simulink model "generic"  (R2022b)
settings: Solver=ode45  StartTime=0.0  StopTime=inf  RelTol=1e-3  EnableMultiTasking=on
values from neighbouring files (symbols this model uses):
  A = cell2mat(A_cell)    [MPCController1.m]    (also in MPC_Fmincon.m)
  B = cell2mat(B_cell)    [MPCController1.m]    (also in MPC_Fmincon.m)
  brake_select = ones(length(speed), length(steering_angle))    [TwoDLook_uptable.m]
  curvature = 0.000:0.001:1    [TwoDLook_uptable.m]
  m = 1600    [MPCController1.m]    (also in MPCController2.m; MPC_Fmincon.m)
  speed = 0:0.1:100    [TwoDLook_uptable.m]
undefined symbols (not defined in the file or in its folder): Amplifier, DiscIntNeverNeededParam, K_d_yawrate, K_dsteering, k_speed, k_stanley, kd, ki, kp, path_curvature
libraries: CarMaker4SL x97, simulink x6, cstblocks x6, simulink_extras x4, autolibshared x1, mpcadaslib x1
(part 6 of 6)

== matlab function generic/CarMaker/VehicleControl/CreateBus VhclCtrl1/Stanley steering & speed//Brake controller/Road sensor set & path planning/Road sensor set & path planning/A* star path planning/getInstantaneousPath Function ==
  data: generated_path input; lookahead_distance input; current_position input; instantaneous_points output; current_heading input
function instantaneous_points = getInstantaneousPoint(generated_path, lookahead_distance, current_position, current_heading)
    % Parameters
    num_points = size(generated_path, 2);
    rotated_point = zeros(1,2);
    instantaneous_point= zeros(1,2);
    disp(generated_path)
    % Find the closest point on the generated path to the current position
    distances = sqrt((generated_path(1, :) - current_position(1)).^2 + (generated_path(2, :) - current_position(2)).^2);
    [~, closest_point_index] = min(distances);
     % Extract the last point along the path based on lookahead distance
    cumulative_distances = cumsum(sqrt(diff(generated_path(1, :)).^2 + diff(generated_path(2, :)).^2));
     % Check if cumulative_distances is non-empty
    if all(cumulative_distances == 0)
        % If there is only one point in the path, use that point
        lookahead_index = closest_point_index;
    else
        % Otherwise, find the index based on lookahead distance
        lookahead_index = closest_point_index + find(cumulative_distances >= lookahead_distance, 1, 'first');
    end
    disp(lookahead_index)
    disp('333')
    
    % Ensure lookahead_index is within valid range
    lookahead_index = min(lookahead_index, num_points);
    
    % Extract the last point from the path
    instantaneous_point = generated_path(:, lookahead_index);
    
    % Transform the point to the vehicle's local coordinate system
    delta_x = instantaneous_point(1) - current_position(1);
    delta_y = instantaneous_point(2) - current_position(2);
    
    rotated_point = [cos(-current_heading) -sin(-current_heading); sin(-current_heading) cos(-current_heading)] * [delta_x; delta_y];
    
    % Adjust the rotated point to be relative to the current position
    instantaneous_points = [current_position(1) + rotated_point(1) current_position(2) + rotated_point(2)];
end

== matlab function generic/CarMaker/VehicleControl/CreateBus VhclCtrl1/Stanley steering & speed//Brake controller/Road sensor set & path planning/Road sensor set & path planning/Dijkestra path planning/getInstantaneousPath Function ==
  data: generated_path input; lookahead_distance input; current_position input; instantaneous_points output; current_heading input
function instantaneous_points = getInstantaneousPoint(generated_path, lookahead_distance, current_position, current_heading)
    % Parameters
    num_points = size(generated_path, 2);
    rotated_point = zeros(1,2);
    instantaneous_point= zeros(1,2);
    disp(generated_path)
    % Find the closest point on the generated path to the current position
    distances = sqrt((generated_path(1, :) - current_position(1)).^2 + (generated_path(2, :) - current_position(2)).^2);
    [~, closest_point_index] = min(distances);
     % Extract the last point along the path based on lookahead distance
    cumulative_distances = cumsum(sqrt(diff(generated_path(1, :)).^2 + diff(generated_path(2, :)).^2));
     % Check if cumulative_distances is non-empty
    if all(cumulative_distances == 0)
        % If there is only one point in the path, use that point
        lookahead_index = closest_point_index;
    else
        % Otherwise, find the index based on lookahead distance
        lookahead_index = closest_point_index + find(cumulative_distances >= lookahead_distance, 1, 'first');
    end
    disp(lookahead_index)
    disp('333')
    
    % Ensure lookahead_index is within valid range
    lookahead_index = min(lookahead_index, num_points);
    
    % Extract the last point from the path
    instantaneous_point = generated_path(:, lookahead_index);
    
    % Transform the point to the vehicle's local coordinate system
    delta_x = instantaneous_point(1) - current_position(1);
    delta_y = instantaneous_point(2) - current_position(2);
    
    rotated_point = [cos(-current_heading) -sin(-current_heading); sin(-current_heading) cos(-current_heading)] * [delta_x; delta_y];
    
    % Adjust the rotated point to be relative to the current position
    instantaneous_points = [current_position(1) + rotated_point(1) current_position(2) + rotated_point(2)];
end

== matlab function generic/CarMaker/VehicleControl/CreateBus VhclCtrl1/Stanley steering & speed//Brake controller/Stanley_controller_with_thottle_and_brake_commands/Stanley steering + PID speed controller/Speed_controller/advancedPID_speed_and_brake_control ==
  settings: updateMethod=DISCRETE
  data: path_curv input; throttle output; min_s_speed input; brake_cmd output; speed_act input; desired_speed input; Kd_speed input; Ki_speed input; Kp_speed input
function [throttle, brake_cmd] = advanced_speed_and_brake_control(path_curv, min_s_speed, speed_act, desired_speed,Kd_speed,Ki_speed,Kp_speed)
    persistent integrator_speed;
    persistent prev_speed_error;
    persistent integrator_brake;
    persistent prev_brake_error;

    if isempty(integrator_speed)
        integrator_speed = 0;
        prev_speed_error = 0;
        integrator_brake = 0;
        prev_brake_error = 0;
    end


   
    % Speed Control (PID)
    %disp(speed_act)
    %disp("teh speed is ")
    %disp(desired_speed)
    speed_error = desired_speed - speed_act;
    %Kp_speed = 1.900;
    %Ki_speed = 0.0300;
    %Kd_speed = 1.00;
    integrator_speed = integrator_speed + speed_error;
    derivative_speed = speed_error - prev_speed_error;
    
    throttle = Kp_speed * speed_error + Ki_speed * integrator_speed + Kd_speed * derivative_speed;

    % Braking Control (PID)
    brake_error = -speed_error;
    Kp_brake = 0.05;
    Ki_brake = 0.01;
    Kd_brake = 0.05;
    integrator_brake = integrator_brake + brake_error;
    derivative_brake = brake_error - prev_brake_error;
    brake_cmd = Kp_brake * brake_error + Ki_brake * integrator_brake + Kd_brake * derivative_brake;

    % Predictive Braking based on Path Curvature
    path_curvature = max(path_curv);
    min_safe_speed = max(min_s_speed);
    predictive_brake_factor = speed_act/100;
    if path_curvature > 0 && speed_act < min_safe_speed
        brake_cmd = brake_cmd + predictive_brake_factor * (min_safe_speed - speed_act);
    end
    % Update persistent variables
    prev_speed_error = speed_error;
    prev_brake_error = brake_error;
end

== matlab function generic/CarMaker/VehicleControl/CreateBus VhclCtrl1/Stanley steering & speed//Brake controller/Stanley_controller_with_thottle_and_brake_commands/MPCLongitudianl_contorl/Speed_regulator/MATLAB Function ==
  data: speed input; braking_distance output; others output
function [braking_distance,others]= calculateBrakingDistance(speed)
    % Estimate the braking distance
        max_deceleration = 5.0;
        safety_factor = 1.5;
        braking_distance = (speed^2) / (2 * max_deceleration) * safety_factor;
        others = speed^2 *3.6/(250*1)* safety_factor*2.2;
end

== matlab function generic/CarMaker/VehicleControl/CreateBus VhclCtrl1/MPC_steering_controllers/Subsystem/MATLAB Function2 ==
  data: heading_error input; dt input; yaw_angle input; yaw_rate input; vx input; delta output; vy input; reference_trajectory input; x input; u input
function delta = adaptive_steering_mpc( heading_error,dt,yaw_angle,yaw_rate, vx, vy, reference_trajectory,x,u)
    % Adaptive Model Predictive Controller (Adaptive MPC) for steering control
    function [c, ceq] = nonlinear_constraints(u, x, vx, dt)
    % Extract control input
    %steering_angle = u(1);
    longitudinal_velocity = u(2);

        % Calculate the next state based on the system dynamics
        x_next = calculate_dynamics(x, u, m, cf, cr, lf, lr, dt, vx);
    
        % Enforce constraints
        c1 = x_next(1) - x(1) - vx * cos(x(4)) * dt;  % Constraint for x position
        c2 = x_next(2) - x(2) - vx * sin(x(4)) * dt;  % Constraint for y position
        
        c3 = x_next(4) - x(4) - longitudinal_velocity * dt;  % Constraint for yaw angle
        c4 = -x(2) - vx * sin(x(4)) * dt;  % Ensure lateral position is within bounds
    
        % Combine inequality constraints
        c = [c1; c2; c3; c4];
    
        % No equality constraints (ceq = 0)
        ceq = [];
    end
        function J = cost_function(u, x, Q, R, N, dt, m, cf, cr, lf, lr, vx, vy)
        % Cost function for fmincon
        x_pred = predict_states(x, u, m, cf, cr, lf, lr, dt, N, vx);
        J = (x_pred - reference_state)' * Q * (x_pred - reference_state) + u' * R * u;
        
    end

    function x_pred = predict_states(x, u, m, cf, cr, lf, lr, dt, N, vx)
        % Predict future states using the model
        A = calculate_A(x, u, m, cf, cr, lf, lr, vx);
        B = calculate_B(x, u, m, cf, cr, lf, lr, vx);

        x_pred = x;
        for i = 1:N
            x_pred = x_pred + A * x_pred * dt + B * u * dt;
        end
    end

    function A = calculate_A(x, u, m, cf, cr, lf, lr, vx)
        % Calculate state matrix A
        A = [-((cf + cr) / (m * vx)), -vx - ((cf * lf - cr * lr) / (m * vx^2)), 0, 0;
             -((cf * lf - cr * lr) / (m * vx)), -((cf * lf^2 + cr * lr^2) / (m * vx^2)), 0, 0;
             1, 0, 0, vx;
             0, 1, vx, 0];
    end

    function B = calculate_B(x, u, m, cf, cr, lf, lr, vx)
        % Calculate input matrix B
        B = [2 * cf / m, 0;
             2 * cf * lf / (m * vx), 0;
             0, 1;
             0, (2 * lf * cf - 2 * lr * cr) / (m * vx)];
    end

    function x_next = calculate_dynamics(x, u, m, cf, cr, lf, lr, dt, vx)
        % Calculate next state using the model
        A = calculate_A(x, u, m, cf, cr, lf, lr, vx);
        B = calculate_B(x, u, m, cf, cr, lf, lr, vx);

        x_next = x + (A * x + B * u) * dt;
    end
    % Define MPC parameters (modify as needed)
    N = 5;  % Prediction horizon
    Q = diag([1, 1, 1, 1]);  % State cost matrix (including heading error)
    R = diag([0.1, 0.1]);  % Input cost matrix

    % Define system parameters (replace these with your actual vehicle parameters)
    m = 1600;           % Vehicle mass [kg]
    l = 2.975;          % Wheelbase [m]
    Iz = 2986.624;      % Vehicle inertia [kg*m^2]
    cf = 80000;         % Front tire cornering stiffness [N/rad]
    cr = 120000;        % Rear tire cornering stiffness [N/rad]
    lf = 1.5;           % Distance from center of gravity to front axle [m]
    lr = 1.475;         % Distance from center of gravity to rear axle [m]

    % Adaptive parameters
    alpha = 0.1;  % Adaptation rate
    theta = [0.1; 0.1];  % Initial guess of parameters

    % State vector (simplified, assuming heading_error is the heading error)
    x = [heading_error; 0; 0; 0];  % Adding lateral error and lateral velocity to the state vector


    % Reference trajectory
    %reference_index = 1;  % Choose the appropriate index for the current time step
    % Extract x and y positions from the trajectory at the chosen index
    x_position = reference_trajectory(1,:);
    y_position = reference_trajectory(2,:);
    % Construct the reference_state vector
    reference_state = [y_position; yaw_angle; vy; yaw_rate];

    % Define cost and constraints for fmincon
    costFunction = @(u) cost_function(u, x, Q, R, N, dt, m, cf, cr, lf, lr, vx, vy);
    lb = [-1.6; -30];  % Lower bounds on steering input and longitudinal velocity change
    ub = [1.6; 30];    % Upper bounds on steering input and longitudinal velocity change
    u0 = [0.1; 0.1];  % Initial guess
    nonlcon = @(u) nonlinear_constraints(u, x, vx, dt);
    % Solve optimization problem to get optimal steering input
    options = optimoptions('fmincon', 'Display', 'off', 'Algorithm', 'sqp');
    %u_opt = fmincon(costFunction, u0, [], [], [], [], lb, ub, [], options);
    disp(reference_state)
    disp(cost_function(u, x, Q, R, N, dt, m, cf, cr, lf, lr, vx, vy))
    u_opt = fmincon(costFunction, u0, [], [], [], [], lb, ub, nonlcon, options);
    % Extract control input (steering angle and longitudinal velocity change)
    delta = u_opt(1);

    % Update adaptive parameters online (using a simple gradient descent)
    %x_next = calculate_dynamics(x, u_opt, m, cf, cr, lf, lr, dt, vx, vy);
    %theta = theta - alpha * (x_next - x) * x';


end

== matlab function generic/CarMaker/VehicleControl/CreateBus VhclCtrl1/MPC_steering_controllers/Subsystem/MATLAB Function6 ==
  data: current_heading input; dt input; vx input; delta output; vy input
function delta = adaptive_steering_mpc(current_heading, dt, vx, vy)
    % Adaptive Model Predictive Controller (Adaptive MPC) for steering control
    persistent model_params theta
        
    function params = initialize_model_params(m, lf, lr, Iz)
        % Initialize model parameters
        % Define the state-space model
        A = [-2 * (lf + lr) / (m * vx), -vx - 2 * (lf * cf - lr * cr) / (m * vx);
             -2 * (lf * cf - lr * cr) / Iz, -2 * (lf^2 * cf + lr^2 * cr) / Iz];
    
        B = [2 * cf / m; 2 * lf * cf / Iz];
    
        % Store parameters in a struct
        params.A = A;
        params.B = B;
    end
    
    function dx = calculate_dynamics(u, params, vx, vy)
        % Calculate the dynamics of the system (Bicycle Model)
    
        % Unpack state variables
        vy1 = vy - params.B(2) * u;  % Correct lateral velocity for the tire slip angle
    
        % Bicycle model equations
        a = (2 * (u - vy1)) / (params.A(1, 2) * vx);
        b = (2 * lf * (u - vy1)) / params.A(2, 2);
    
        % State dynamics
        dx1 = a * dt;
        dx2 = b * dt;
    
        % Update state variables
        dx = [dx1; dx2];
    end

    % Define Q and R matrices
    Q = eye(2);  % Weighting matrix for state
    R = eye(1);  % Weighting matrix for control input

    % Define system parameters (replace these with your actual vehicle parameters)
    m = 1600;           % Vehicle mass [kg]
    l = 2.975;          % Wheelbase [m]
    Iz = 2986.624;      % Vehicle inertia [kg*m^2]
    cf = 80000;         % Front tire cornering stiffness [N/rad]
    cr = 120000;        % Rear tire cornering stiffness [N/rad]
    lf = 1.5;           % Distance from center of gravity to front axle [m]
    lr = 1.475;         % Distance from center of gravity to rear axle [m]

    % Adaptive parameters
    alpha = 0.1;  % Adaptation rate

    % Update the model parameters if not initialized
    if isempty(model_params)
        model_params = initialize_model_params(m, lf, lr, Iz);
    end

    % Update adaptive parameters if not initialized
    if isempty(theta)
        theta = [0.1; 0.1];  % Initial guess of parameters
    end

    % State vector (simplified, assuming current_heading is the heading error)
    x = [current_heading; 0];

    % Define matrices for quadprog
    H = blkdiag(Q, R);
    f = zeros(size(H, 1), 1);

    % Define linear inequality constraints for quadprog
    Aineq = [];
    Bineq = [];
    % Define linear equality constraints for quadprog
    Aeq = [];
    Beq = [];
    % Define lower and upper bounds for quadprog
    lb = [-1.6; -1.6; -1.6];  % Lower bounds on steering input for each dimension
    ub = [1.6; 1.6; 1.6];     % Upper bounds on steering input for each dimension


    % Initial guess for the control input
    u0 = zeros(size(H, 2), 1);  % Initialize u0 with the correct size

    % Solve the quadratic programming problem with quadprog
    options = optimoptions('quadprog', 'Display', 'off','Algorithm','active-set');
    [u_opt, ~, exitflag] = quadprog(H, f, Aineq, Bineq, Aeq, Beq, lb, ub, u0, options);

    % Check if optimization was successful
    if exitflag <= 0
        error('Quadprog failed to converge. Consider adjusting the problem formulation or solver options.');
    end

    % Update adaptive parameters online (using a simple gradient descent)
    %x_next = x + calculate_dynamics(u_opt, model_params, vx, vy);
    %theta = theta - alpha * (x_next - (x + calculate_dynamics(u_opt, model_params, vx, vy))) * x';

    % Extract control input (steering angle) from the optimization result
    delta = u_opt;
end

== matlab function generic/CarMaker/VehicleControl/CreateBus VhclCtrl1/MPC_steering_controllers/Subsystem/MATLAB Function7 ==
  data: u input; dt input; vx input; delta output; vy input; cr input; cf input; yaw input; dx output; dx1 output
function [delta,dx,dx1] = adaptive_steering_mpc(u, dt, vx, vy,cr,cf,yaw)
    % Adaptive Model Predictive Controller (Adaptive MPC) for steering control
   % persistent model_params theta
    % Define Q and R matrices
    Q = eye(2);  % Weighting matrix for state
    R = eye(1);  % Weighting matrix for control input

    % Define system parameters (replace these with your actual vehicle parameters)
    m = 1600;           % Vehicle mass [kg]
    l = 2.975;          % Wheelbase [m]
    Iz = 2986.624;      % Vehicle inertia [kg*m^2]
    %cf = 80000;         % Front tire cornering stiffness [N/rad]
    %cr = 120000;        % Rear tire cornering stiffness [N/rad]
    lf = 1.488;           % Distance from center of gravity to front axle [m]
    lr = -1.487;         % Distance from center of gravity to rear axle [m]
    if vx<0.5
        vx = 0.5;
    end
    function params = initialize_model_params(Iz,m,vx,cf,cr ,lf, lr)
        % Initialize model parameters
        % Define the state-space model
        A = [-(cr + cf) / (m * vx), -(lf * cf - lr * cr) / (m * vx)+vx^2;
             -(lf * cf - lr * cr) / (Iz*vx), -(lf^2 * cf + lr^2 * cr) / (Iz*vx)];
    
        B = [cf / m, cr/m; lf * cf / Iz, -lr*cr/Iz];
    
        % Store parameters in a struct
        params.A = A;
        params.B = B;
    end
    
    function [dx,dx1] = calculate_dynamics(params, yaw, vy,lf,dt,u)
        % Calculate the dynamics of the system (Bicycle Model)
    
        % Unpack state variables
        vy1 = vy - params.B(2) * u(1);  % Correct lateral velocity for the tire slip angle
        %vy1 = params.B(2);
        % Bicycle model equations
        %a = (2 * (u(1) - vy1)) / (params.A(1, 2) * vx);
        %b = (2 * lf * (u(2) - vy1)) / params.A(2, 2);
        % State dynamics
        %dx1 = a * dt;
        %dx2 = b * dt;
        dx1 = params.B *[0;u(2)]*dt;
        x_dot = params.A *[vy1;yaw]*dt+params.B *[0;u(2)]*dt;
        % Update state variables
        dx =x_dot; %[dx1; dx2];
    end
    params = initialize_model_params(Iz,m,vx,cf,cr ,lf, lr);
    [dx,dx1] = calculate_dynamics(params, yaw, vy,lf,dt,u);
    delta = atan(dx(2)*l/(vx*(1+ (-0.01*vx))));

%     % Adaptive parameters
%     alpha = 0.1;  % Adaptation rate
% 
%     % Update the model parameters if not initialized
%     if isempty(model_params)
%         model_params = initialize_model_params(m, lf, lr, Iz);
%     end
% 
%     % Update adaptive parameters if not initialized
%     if isempty(theta)
%         theta = [0.1; 0.1];  % Initial guess of parameters
%     end
% 
%     % State vector (simplified, assuming current_heading is the heading error)
%     x = [current_heading; 0];
% 
%     % Define matrices for quadprog
%     H = blkdiag(Q, R);
%     f = zeros(size(H, 1), 1);
% 
%     % Define linear inequality constraints for quadprog
%     Aineq = [];
%     Bineq = [];
%     % Define linear equality constraints for quadprog
%     Aeq = [];
%     Beq = [];
%     % Define lower and upper bounds for quadprog
%     lb = [-1.6; -1.6; -1.6];  % Lower bounds on steering input for each dimension
%     ub = [1.6; 1.6; 1.6];     % Upper bounds on steering input for each dimension
% 
% 
%     % Initial guess for the control input
%     u0 = zeros(size(H, 2), 1);  % Initialize u0 with the correct size
% 
%     % Solve the quadratic programming problem with quadprog
%     options = optimoptions('quadprog', 'Display', 'off','Algorithm','active-set');
%     [u_opt, ~, exitflag] = quadprog(H, f, Aineq, Bineq, Aeq, Beq, lb, ub, u0, options);
% 
%     % Check if optimization was successful
%     if exitflag <= 0
%         error('Quadprog failed to converge. Consider adjusting the problem formulation or solver options.');
%     end
% 
%     % Update adaptive parameters online (using a simple gradient descent)
%     %x_next = x + calculate_dynamics(u_opt, model_params, vx, vy);
%     %theta = theta - alpha * (x_next - (x + calculate_dynamics(u_opt, model_params, vx, vy))) * x';
% 
%     % Extract control input (steering angle) from the optimization result
%     delta = u_opt;
end

== matlab function generic/CarMaker/VehicleControl/CreateBus VhclCtrl1/MPC_steering_controllers/Tradition_MPC/MPC_steering_control ==
  data: Lateral_deviation input; steering_cmd output; A input; B input
function steering_cmd = MPC_Steering_control(Lateral_deviation,A,B)
    % Model Predictive Controller (MPC) for speed contol
    %speed_ref  = speed_rf+0.4;
    %Lateral_deviation= current_speed - speed_ref;
    % Define MPC parameters
    Ts = 0.1;  % Sampling time
    N = 10;    % Prediction horizon
    Q = 1;     % State weight
    R = 1;     % Input weight
    S = 0.1;   % Terminal state weight (integral term)
    
    % State-space model (simplified for illustration)
    %A = 0.8;
    %B = Ts;
    
    % Define cost and constraints for fmincon
    costFunction = @(u) (Lateral_deviation + B * u)' * Q * (Lateral_deviation + B * u) + u' * R * u + S * sum(u);
    Aeq = [];
    Beq = [];
    Aineq = [];
    Bineq = [];
    lb = -1.6; % Lower bound on throttle_Brake
    ub = 1.6;  % Upper bound on throttle_Brake
    
    % Steady-state error constraint
    Aineq = [Aineq; B];
    Bineq = [Bineq; -Lateral_deviation];
    
    % Initial guess
    u0 = 0;
    
    % Solve optimization problem
    options = optimoptions('fmincon', 'Display', 'off', 'Algorithm', 'sqp');
    u_opt = fmincon(costFunction, u0, Aineq, Bineq, Aeq, Beq, lb, ub, [], options);
    
    % Extract control input (throttle_Brake) from the optimization result
    steering_cmd = u_opt;
end

== matlab function generic/CarMaker/VehicleControl/CreateBus VhclCtrl1/MPC_steering_controllers/Tradition_MPC/MPC_steering_control1 ==
  data: Heading_error input; steering_cmd output; A input; B input
function steering_cmd = MPC_Steering_control(Heading_error,A,B)
    % Model Predictive Controller (MPC) for speed contol
    %speed_ref  = speed_rf+0.4;
    %Heading_error= current_speed - speed_ref;
    % Define MPC parameters
    Ts = 0.1;  % Sampling time
    N = 10;    % Prediction horizon
    Q = 1;     % State weight
    R = 1;     % Input weight
    S = 0.1;   % Terminal state weight (integral term)
    
    % State-space model (simplified for illustration)
    %A = 0.8;
    %B = Ts;
    
    % Define cost and constraints for fmincon
    costFunction = @(u) (Heading_error + B * u)' * Q * (Heading_error + B * u) + u' * R * u + S * sum(u);
    Aeq = [];
    Beq = [];
    Aineq = [];
    Bineq = [];
    lb = -1.6; % Lower bound on throttle_Brake
    ub = 1.6;  % Upper bound on throttle_Brake
    
    % Steady-state error constraint
    Aineq = [Aineq; B];
    Bineq = [Bineq; -Heading_error];
    
    % Initial guess
    u0 = 0;
    
    % Solve optimization problem
    options = optimoptions('fmincon', 'Display', 'off', 'Algorithm', 'sqp');
    u_opt = fmincon(costFunction, u0, Aineq, Bineq, Aeq, Beq, lb, ub, [], options);
    
    % Extract control input (throttle_Brake) from the optimization result
    steering_cmd = u_opt;
end

== matlab function generic/CarMaker/VehicleControl/CreateBus VhclCtrl1/Stanley steering & speed//Brake controller/Stanley_controller_with_thottle_and_brake_commands/MPCLongitudianl_contorl/MPC_speed_control ==
  data: speed_error input; throttle_Brake output; A input; B input
function throttle_Brake = MPC_speed_control(speed_error,A,B)
    % Model Predictive Controller (MPC) for speed contol
    %speed_ref  = speed_rf+0.4;
    %speed_error= current_speed - speed_ref;
    % Define MPC parameters
    Ts = 0.1;  % Sampling time
    N = 10;    % Prediction horizon
    Q = 1;     % State weight
    R = 1;     % Input weight
    S = 0.1;   % Terminal state weight (integral term)
    
    % State-space model (simplified for illustration)
    %A = 0.8;
    %B = Ts;
    
    % Define cost and constraints for fmincon
    costFunction = @(u) (speed_error + B * u)' * Q * (speed_error + B * u) + u' * R * u + S * sum(u);
    Aeq = [];
    Beq = [];
    Aineq = [];
    Bineq = [];
    lb = 0; % Lower bound on throttle_Brake
    ub = 1;  % Upper bound on throttle_Brake
    
    % Steady-state error constraint
    Aineq = [Aineq; B];
    Bineq = [Bineq; -speed_error];
    
    % Initial guess
    u0 = 0;
    
    % Solve optimization problem
    options = optimoptions('fmincon', 'Display', 'off', 'Algorithm', 'sqp');
    u_opt = fmincon(costFunction, u0, Aineq, Bineq, Aeq, Beq, lb, ub, [], options);
    
    % Extract control input (throttle_Brake) from the optimization result
    throttle_Brake = u_opt;
end

== matlab function generic/CarMaker/VehicleControl/CreateBus VhclCtrl1/Stanley steering & speed//Brake controller/Stanley controller with path_planning/Stanley controller with path_planning/MATLAB Function ==
  data: path input; dev input; e output; yaw input; speed_act input; err_fr_axle output; cross_track_steering output; heading_err output; steering output
function [e, err_fr_axle, cross_track_steering, heading_err, steering]  = conversion(path,dev,yaw,speed_act)
%path = [path_x;path_y];
function distance = calc_distance(pt,v1,v2)
    vect = v1 - v2;
    p_to_vect = pt - v2;
    crossVP = cross(vect,p_to_vect);
    distance = norm(crossVP) / norm(vect) * crossVP(3)/abs(crossVP(3));
end

e = zeros(1);
cross_track_steering = zeros(1);
heading_err = zeros(1);
steering=zeros(1);
err_fr_axle = zeros(1);

k_exp = 1.3059;
k = 15.028 + speed_act^k_exp;
k_ref = 2.62;

% path_index = fix(k_path * speed_act);
% if path_index > 13
%     path_index = 13;
% end
% 
% P_prev = path(:,6 + path_index);
% P_next = path(:,7 + path_index);

fr_axle = [-1.488 0 0];
distances = sqrt((path(1,:) - 1.488).^2 + (path(2,:) - 0).^2);
% Find the index of the closest point on the path
[~,err_fr_axle_ind] = min(distances);
if err_fr_axle_ind == 1
    err_fr_axle_ind = 2;
end
err_fr_axle = calc_distance(fr_axle,[path(1,err_fr_axle_ind - 1) path(2,err_fr_axle_ind - 1) 0],[path(1,err_fr_axle_ind) path(2,err_fr_axle_ind) 0]);

B = [-1.488 + k_ref * (speed_act / 27) 0 0];
distances_err = sqrt((path(1,:) - B(1)).^2 + (path(2,:) - 0).^2);
[~,err_ind] = min(distances_err);
if err_ind < 2
    err_ind = 2;
end
error = calc_distance(B,[path(1,err_ind - 1) path(2,err_ind - 1) 0],[path(1,err_ind) path(2,err_ind) 0]);


P_prev = path(:, err_ind-1);
P_next = path(:, err_ind);

x1 = P_prev(1,1);
y1 = P_prev(2,1);
x2 = P_next(1,1);
y2 = P_next(2,1);

a = (y2 - y1)/-(x2 + x1);
b = 1;
%c = -x1 * (y2 - y1) + y1 * (x2 - x1);


if speed_act ~= 0
    %e = c+b*y1/sqrt((a^2)+(b^2));
    e = error;
    
    cross_track_steering = atan(k * e / speed_act);
    heading_err = atan(-a / b) - yaw;
    %heading_err = 1/(tan(-a/b))-yaw;
    steering = heading_err + cross_track_steering;
end
end

== matlab function generic/CarMaker/VehicleControl/CreateBus VhclCtrl1/MPC_steering_controllers/Subsystem/MATLAB Function1 ==
  data: dev input; steering output; B input
function steering = advanced_speed_control_mpc(dev,B)
    % Model Predictive Controller (MPC) for speed contol
    % Define MPC parameters
    Ts = 0.1;  % Sampling time
    N = 10;    % Prediction horizon
    Q = 1;     % State weight
    R = 1;     % Input weight
    S = 0.1;   % Terminal state weight (integral term)
    
    % State-space model (simplified for illustration)
    %A = 0.8;
    %B = Ts;
    
    % Define cost and constraints for fmincon
    costFunction = @(u) (dev + B * u)' * Q * (dev + B * u) + u' * R * u + S * sum(u);
    Aeq = [];
    Beq = [];
    Aineq = [];
    Bineq = [];
    lb = -3.14; % Lower bound on throttle
    ub = 3.14;  % Upper bound on throttle
    
    % Steady-state error constraint
    Aineq = [Aineq; B];
    Bineq = [Bineq; -dev];
    
    % Initial guess
    u0 = 0;
    
    % Solve optimization problem
    options = optimoptions('fmincon', 'Display', 'off', 'Algorithm', 'sqp');
    u_opt = fmincon(costFunction, u0, Aineq, Bineq, Aeq, Beq, lb, ub, [], options);
    
    % Extract control input (throttle) from the optimization result
    steering = u_opt;
end

== matlab function generic/CarMaker/VehicleControl/CreateBus VhclCtrl1/Stanley steering & speed//Brake controller/Stanley_controller_with_thottle_and_brake_commands/Stanley steering + PID speed controller/Speed_controller/calculate_path_curvature ==
  data: path input; path_curvature output size=[1 20]; min_safe_speed output size=[1 20]; velocity_y input; velocity_x input; steering_angel input
function [path_curvature, min_safe_speed] = calculate_path_curvature(path,velocity_y,velocity_x,steering_angel)
    v_x = velocity_x* ones(1,20);
    v_y = velocity_y*ones(1,20);
    x = path(1,:)+v_x;
    y = path(2,:)+v_y;
    % First and second derivatives
    dx = gradient(x);
    dy = gradient(y);
    
    ddx = gradient(dx);
    ddy = gradient(dy);
    
    % Path curvature
    path_curvature = (dx .* ddy - dy .* ddx) ./ (dx.^2 + dy.^2).^(3/2);
    R = sqrt(1.61^2 +(1.61+1.28)^2*cot(steering_angel)^2)/12;
    % Minimum safe speed
    g = 9.81; % gravitational acceleration
    if max(path_curvature)>0.001 || max(path_curvature)<-0.001

        min_safe_speed = sqrt(g ./ abs(path_curvature));
    else
        min_safe_speed = sqrt(g .* abs(path_curvature));
end

== matlab function generic/CarMaker/VehicleControl/CreateBus VhclCtrl1/Stanley steering & speed//Brake controller/Stanley_controller_with_thottle_and_brake_commands/Stanley steering + PID speed controller/Stanely_controller ==
  data: dev_angle input; dev input; x1 input; x2 input; y1 input; y2 input; speed_act input; e output; cross_track_steering output; steering output
function [e, cross_track_steering, steering]  = conversion(dev_angle,dev, x1,x2,y1,y2,speed_act)


e = zeros(1);
cross_track_steering = zeros(1);


k_exp = 1.36;
k_def = 6;
k = k_def + abs(speed_act)^k_exp;

% Perform linear regression to find a, b, and c
% X = [path(1, :); path(2, :); ones(1, 20)]';  % Create a matrix for linear regression
% coefficients = X \ -1 * ones(20, 1);
% 
% % Extract the coefficients a, b, and c
% a = coefficients(1);
% b = coefficients(2);
% c = coefficients(3);
if (x2 ==0 && x1 ==0)|| x2==x1
a = 0;
b = 1;
c = y2+a*x2;
else
a = -(y2 - y1)/(x2-x1);
b = 1;
c = y2+a*x2;
end

if speed_act ~=0
    %e =abs(a*x_car+b*y_car+c)\sqrt(a^2+b^2); %abs(Dev_dis);
    e =-1*dev;% deviation distance
    cross_track_steering = atan(e*k / (1+speed_act));
    %heading_err = atan(-a/b)-yaw;
    heading_err = dev_angle; % heading error OR deviation angle
    steering = heading_err + cross_track_steering;

else
    steering = 0;
end
end
